simulink model "Super2"  (Simulink 8.7)
settings: Solver=ode45  StartTime=0.0  StopTime=10.0  RelTol=1e-3
settings Model: Creator=scaife  LastModifiedBy=bourbouh  ExtModeAutoUpdateStatusClock=off
settings DataIOCC: SignalLoggingSaveFormat=ModelDataLogs  SignalLoggingName=sigsOut
settings DebuggingCC: SaveWithParameterizedLinksMsg=none  SignalResolutionControl=TryResolveAllWithWarning  MultiTaskDSMMsg=warning  MultiTaskCondExecSysMsg=none
settings HardwareCC: TargetUnknown=on
settings SFSimCC: SimParseCustomCode=off
settings GRTTargetCC: GeneratePreprocessorConditionals=Use local settings  CombineOutputUpdateFcns=off  GRTInterface=on

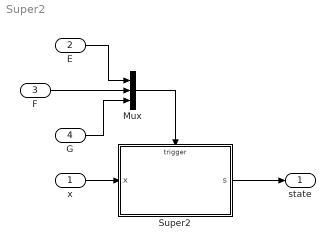
== system Super2 ==
  x : Inport
  E : Inport  Port=2
  F : Inport  Port=3
  G : Inport  Port=4
  Mux : Mux  Inputs=3
  Super2 : Stateflow chart  TreatAsAtomicUnit=on
  state : Outport
  wires:
  E/1 -> Mux/1
  F/1 -> Mux/2
  G/1 -> Mux/3
  x/1 -> Super2/1(x)
  Mux/1 -> Super2/Trigger
  Super2/1(s) -> state/1

== stateflow chart Super2 ==
  state A
    en: s = 1
  state B
    en: s = 3
  state C
    state C1
      en: s = 2
    (default) -> C1
  A -> C [order 1] : F
  C -> B : F
  (default) -> A
  C1 -> B : E
  A -> C1 [order 2] : E
  B -> A : G
  data: x input int32; s output double
  events: E input EITHER_EDGE_EVENT; F input EITHER_EDGE_EVENT; G input EITHER_EDGE_EVENT
